simulink model "kamerol"  (R2021b)
settings: Solver=VariableStepAuto  StartTime=0.0  StopTime=10.0  RelTol=1e-3
undefined symbols (not defined in the file): admireDB
libraries: simulink_extras x104, simulink x24, sharedutil x1
(part 13 of 14)

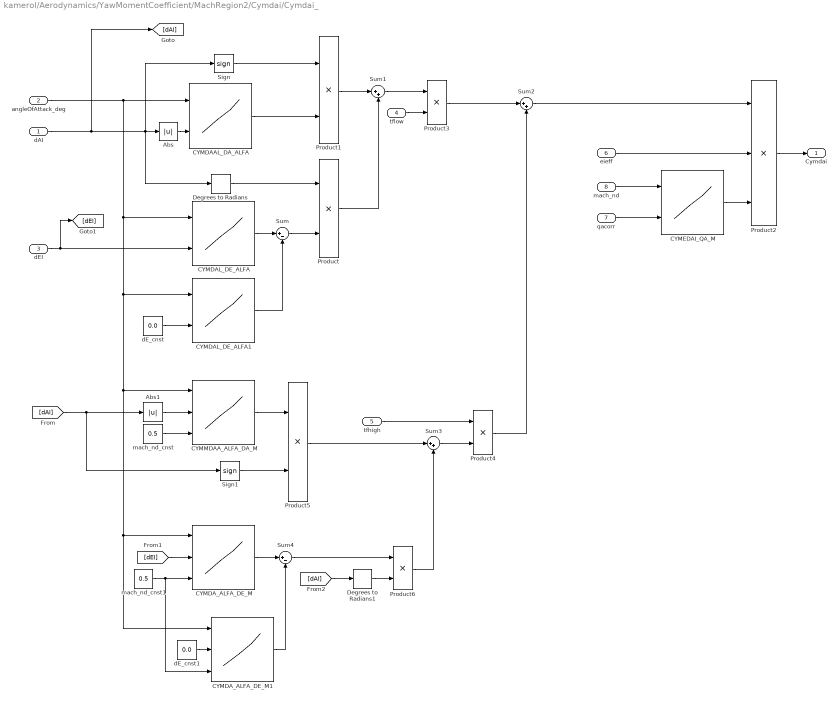
== system kamerol/Aerodynamics/YawMomentCoefficient/MachRegion2/Cymdai/Cymdai_ ==
  dAI : Inport
  angleOfAttack_deg : Inport  Port=2
  dEI : Inport  Port=3
  tflow : Inport  Port=4
  tfhigh : Inport  Port=5
  eieff : Inport  Port=6
  qacorr : Inport  Port=7
  mach_nd : Inport  Port=8
  Abs : Abs
  Abs1 : Abs
  CYMDAAL_DA_ALFA : Lookup_n-D  BreakpointsForDimension1=admireDB.aerodata_asym_ext.CYMDAAL.breakpoints.ALFA  BreakpointsForDimension2=admireDB.aerodata_asym_ext.CYMDAAL.breakpoints.DA  BreakpointsForDimension3=[5, 7]  Table=admireDB.aerodata_asym_ext.CYMDAAL.newTable  ExtrapMethod=Clip  InternalRulePriority=Speed  RndMeth=Simplest  InputSameDT=on
      settings: InputPortMap=u0,u1
  CYMDAL_DE_ALFA : Lookup_n-D  BreakpointsForDimension1=admireDB.aerodata_asym_ext.CYMDAL.breakpoints.ALFA  BreakpointsForDimension2=admireDB.aerodata_asym_ext.CYMDAL.breakpoints.DE  BreakpointsForDimension3=[5, 7]  Table=admireDB.aerodata_asym_ext.CYMDAL.newTable  ExtrapMethod=Clip  InternalRulePriority=Speed  RndMeth=Simplest  InputSameDT=on
      settings: InputPortMap=u0,u1
  CYMDAL_DE_ALFA1 : Lookup_n-D  BreakpointsForDimension1=admireDB.aerodata_asym_ext.CYMDAL.breakpoints.ALFA  BreakpointsForDimension2=admireDB.aerodata_asym_ext.CYMDAL.breakpoints.DE  BreakpointsForDimension3=[5, 7]  Table=admireDB.aerodata_asym_ext.CYMDAL.newTable  ExtrapMethod=Clip  InternalRulePriority=Speed  RndMeth=Simplest  InputSameDT=on
      settings: InputPortMap=u0,u1
  CYMDA_ALFA_DE_M : Lookup_n-D  NumberOfTableDimensions=3  BreakpointsForDimension1=admireDB.aerodata_asym_ext.CYMDA.breakpoints.ALFA  BreakpointsForDimension2=admireDB.aerodata_asym_ext.CYMDA.breakpoints.DE  BreakpointsForDimension3=admireDB.aerodata_asym_ext.CYMDA.breakpoints.M  Table=admireDB.aerodata_asym_ext.CYMDA.newTable  ExtrapMethod=Clip  InternalRulePriority=Speed  RndMeth=Simplest  InputSameDT=on
      settings: InputPortMap=u0,u1,u2
  CYMDA_ALFA_DE_M1 : Lookup_n-D  NumberOfTableDimensions=3  BreakpointsForDimension1=admireDB.aerodata_asym_ext.CYMDA.breakpoints.ALFA  BreakpointsForDimension2=admireDB.aerodata_asym_ext.CYMDA.breakpoints.DE  BreakpointsForDimension3=admireDB.aerodata_asym_ext.CYMDA.breakpoints.M  Table=admireDB.aerodata_asym_ext.CYMDA.newTable  ExtrapMethod=Clip  InternalRulePriority=Speed  RndMeth=Simplest  InputSameDT=on
      settings: InputPortMap=u0,u1,u2
  CYMEDAI_QA_M : Lookup_n-D  BreakpointsForDimension1=admireDB.aerodata_asym_ext.CYMEDAI.breakpoints.M  BreakpointsForDimension2=admireDB.aerodata_asym_ext.CYMEDAI.breakpoints.QA  BreakpointsForDimension3=[5, 7]  Table=admireDB.aerodata_asym_ext.CYMEDAI.newTable  ExtrapMethod=Clip  InternalRulePriority=Speed  RndMeth=Simplest  InputSameDT=on
      settings: InputPortMap=u0,u1
  CYMMDAA_ALFA_DA_M : Lookup_n-D  NumberOfTableDimensions=3  BreakpointsForDimension1=admireDB.aerodata_asym_ext.CYMMDAA.breakpoints.ALFA  BreakpointsForDimension2=admireDB.aerodata_asym_ext.CYMMDAA.breakpoints.DA  BreakpointsForDimension3=admireDB.aerodata_asym_ext.CYMMDAA.breakpoints.M  Table=admireDB.aerodata_asym_ext.CYMMDAA.newTable  ExtrapMethod=Clip  InternalRulePriority=Speed  RndMeth=Simplest  InputSameDT=on
      settings: InputPortMap=u0,u1,u2
  Degrees to Radians : simulink_extras/Transformations/Degrees to Radians
  Degrees to Radians1 : simulink_extras/Transformations/Degrees to Radians
  Product{,1,3..4,6} (5 alike) : Product
  Product2 : Product  Inputs=3
  Product5 : Product  Inputs=**
  Sign : Signum
  Sign1 : Signum
  Sum : Sum  Inputs=|+-
  Sum1 : Sum  Inputs=|++
  Sum2 : Sum  Inputs=|++
  Sum3 : Sum  Inputs=|++
  Sum4 : Sum  Inputs=|+-
  dE_cnst : Constant  Value=0.0
  dE_cnst1 : Constant  Value=0.0
  mach_nd_cnst : Constant  Value=0.5
  mach_nd_cnst1 : Constant  Value=0.5
  Cymdai : Outport
  wires:
  Abs1/1 -> CYMMDAA_ALFA_DA_M/2
  CYMEDAI_QA_M/1 -> Product2/3
  mach_nd/1 -> CYMEDAI_QA_M/1
  qacorr/1 -> CYMEDAI_QA_M/2
  eieff/1 -> Product2/2
  Sum1/1 -> Product3/1
  Product/1 -> Sum1/2
  Product1/1 -> Sum1/1
  Sign/1 -> Product1/1
  CYMDAAL_DA_ALFA/1 -> Product1/2
  Degrees to Radians/1 -> Product/1
  Sum/1 -> Product/2
  CYMDAL_DE_ALFA1/1 -> Sum/2
  CYMDAL_DE_ALFA/1 -> Sum/1
  dEI/1 -> CYMDAL_DE_ALFA/2, [dEI]
  dE_cnst/1 -> CYMDAL_DE_ALFA1/2
  Abs/1 -> CYMDAAL_DA_ALFA/2
  dAI/1 -> [dAI], Sign/1, Abs/1, Degrees to Radians/1
  Product2/1 -> Cymdai/1
  tflow/1 -> Product3/2
  Sum2/1 -> Product2/1
  tfhigh/1 -> Product4/1
  Product3/1 -> Sum2/1
  Product4/1 -> Sum2/2
  angleOfAttack_deg/1 -> CYMDAAL_DA_ALFA/1, CYMDAL_DE_ALFA1/1, CYMDA_ALFA_DE_M1/1, CYMDA_ALFA_DE_M/1, CYMMDAA_ALFA_DA_M/1, CYMDAL_DE_ALFA/1
  mach_nd_cnst/1 -> CYMMDAA_ALFA_DA_M/3
  Sign1/1 -> Product5/2
  [dAI] -> Sign1/1, Abs1/1
  CYMMDAA_ALFA_DA_M/1 -> Product5/1
  Product5/1 -> Sum3/1
  mach_nd_cnst1/1 -> CYMDA_ALFA_DE_M/3, CYMDA_ALFA_DE_M1/3
  [dEI] -> CYMDA_ALFA_DE_M/2
  dE_cnst1/1 -> CYMDA_ALFA_DE_M1/2
  CYMDA_ALFA_DE_M/1 -> Sum4/1
  CYMDA_ALFA_DE_M1/1 -> Sum4/2
  Sum4/1 -> Product6/1
  Degrees to Radians1/1 -> Product6/2
  [dAI] -> Degrees to Radians1/1
  Product6/1 -> Sum3/2
  Sum3/1 -> Product4/2

== system kamerol/Aerodynamics/YawMomentCoefficient/MachRegion2/Cymdaib/Cymdaib_ ==
  angleOfAttack_deg : Inport
  dAI : Inport  Port=2
  angleOfSideslip_deg : Inport  Port=3
  eieff : Inport  Port=4
  tflow : Inport  Port=5
  Abs : Abs
  Abs1 : Abs
  Abs2 : Abs
  CYMDABAL_ALFA : Lookup_n-D  NumberOfTableDimensions=1  BreakpointsForDimension1=admireDB.aerodata_asym_ext.CYMDABAL.breakpoints.ALFA  BreakpointsForDimension3=[5, 7]  Table=admireDB.aerodata_asym_ext.CYMDABAL.newTable  ExtrapMethod=Clip  InternalRulePriority=Speed  RndMeth=Simplest  InputSameDT=on
  Constant : Constant  Value=1/30
  Constant1 : Constant  Value=1/20
  Product : Product  Inputs=*******
  Cymdaib : Outport
  wires:
  eieff/1 -> Product/6
  Abs2/1 -> Product/4
  Constant1/1 -> Product/5
  angleOfSideslip_deg/1 -> Abs2/1
  Constant/1 -> Product/3
  Abs1/1 -> Product/2
  Abs/1 -> CYMDABAL_ALFA/1
  dAI/1 -> Abs1/1
  CYMDABAL_ALFA/1 -> Product/1
  angleOfAttack_deg/1 -> Abs/1
  Product/1 -> Cymdaib/1
  tflow/1 -> Product/7

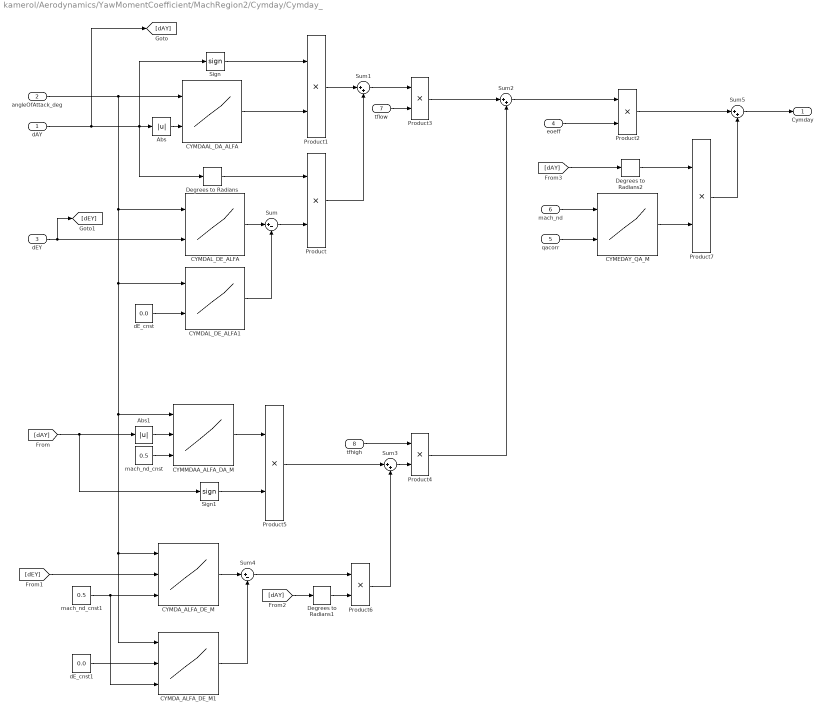
== system kamerol/Aerodynamics/YawMomentCoefficient/MachRegion2/Cymday/Cymday_ ==
  dAY : Inport
  angleOfAttack_deg : Inport  Port=2
  dEY : Inport  Port=3
  eoeff : Inport  Port=4
  qacorr : Inport  Port=5
  mach_nd : Inport  Port=6
  tflow : Inport  Port=7
  tfhigh : Inport  Port=8
  Abs : Abs
  Abs1 : Abs
  CYMDAAL_DA_ALFA : Lookup_n-D  BreakpointsForDimension1=admireDB.aerodata_asym_ext.CYMDAAL.breakpoints.ALFA  BreakpointsForDimension2=admireDB.aerodata_asym_ext.CYMDAAL.breakpoints.DA  BreakpointsForDimension3=[5, 7]  Table=admireDB.aerodata_asym_ext.CYMDAAL.newTable  ExtrapMethod=Clip  InternalRulePriority=Speed  RndMeth=Simplest  InputSameDT=on
      settings: InputPortMap=u0,u1
  CYMDAL_DE_ALFA : Lookup_n-D  BreakpointsForDimension1=admireDB.aerodata_asym_ext.CYMDAL.breakpoints.ALFA  BreakpointsForDimension2=admireDB.aerodata_asym_ext.CYMDAL.breakpoints.DE  BreakpointsForDimension3=[5, 7]  Table=admireDB.aerodata_asym_ext.CYMDAL.newTable  ExtrapMethod=Clip  InternalRulePriority=Speed  RndMeth=Simplest  InputSameDT=on
      settings: InputPortMap=u0,u1
  CYMDAL_DE_ALFA1 : Lookup_n-D  BreakpointsForDimension1=admireDB.aerodata_asym_ext.CYMDAL.breakpoints.ALFA  BreakpointsForDimension2=admireDB.aerodata_asym_ext.CYMDAL.breakpoints.DE  BreakpointsForDimension3=[5, 7]  Table=admireDB.aerodata_asym_ext.CYMDAL.newTable  ExtrapMethod=Clip  InternalRulePriority=Speed  RndMeth=Simplest  InputSameDT=on
      settings: InputPortMap=u0,u1
  CYMDA_ALFA_DE_M : Lookup_n-D  NumberOfTableDimensions=3  BreakpointsForDimension1=admireDB.aerodata_asym_ext.CYMDA.breakpoints.ALFA  BreakpointsForDimension2=admireDB.aerodata_asym_ext.CYMDA.breakpoints.DE  BreakpointsForDimension3=admireDB.aerodata_asym_ext.CYMDA.breakpoints.M  Table=admireDB.aerodata_asym_ext.CYMDA.newTable  ExtrapMethod=Clip  InternalRulePriority=Speed  RndMeth=Simplest  InputSameDT=on
      settings: InputPortMap=u0,u1,u2
  CYMDA_ALFA_DE_M1 : Lookup_n-D  NumberOfTableDimensions=3  BreakpointsForDimension1=admireDB.aerodata_asym_ext.CYMDA.breakpoints.ALFA  BreakpointsForDimension2=admireDB.aerodata_asym_ext.CYMDA.breakpoints.DE  BreakpointsForDimension3=admireDB.aerodata_asym_ext.CYMDA.breakpoints.M  Table=admireDB.aerodata_asym_ext.CYMDA.newTable  ExtrapMethod=Clip  InternalRulePriority=Speed  RndMeth=Simplest  InputSameDT=on
      settings: InputPortMap=u0,u1,u2
  CYMEDAY_QA_M : Lookup_n-D  BreakpointsForDimension1=admireDB.aerodata_asym_ext.CYMEDAY.breakpoints.M  BreakpointsForDimension2=admireDB.aerodata_asym_ext.CYMEDAY.breakpoints.QA  BreakpointsForDimension3=[5, 7]  Table=admireDB.aerodata_asym_ext.CYMEDAY.newTable  ExtrapMethod=Clip  InternalRulePriority=Speed  RndMeth=Simplest  InputSameDT=on
      settings: InputPortMap=u0,u1
  CYMMDAA_ALFA_DA_M : Lookup_n-D  NumberOfTableDimensions=3  BreakpointsForDimension1=admireDB.aerodata_asym_ext.CYMMDAA.breakpoints.ALFA  BreakpointsForDimension2=admireDB.aerodata_asym_ext.CYMMDAA.breakpoints.DA  BreakpointsForDimension3=admireDB.aerodata_asym_ext.CYMMDAA.breakpoints.M  Table=admireDB.aerodata_asym_ext.CYMMDAA.newTable  ExtrapMethod=Clip  InternalRulePriority=Speed  RndMeth=Simplest  InputSameDT=on
      settings: InputPortMap=u0,u1,u2
  Degrees to Radians : simulink_extras/Transformations/Degrees to Radians
  Degrees to Radians1 : simulink_extras/Transformations/Degrees to Radians
  Degrees to Radians2 : simulink_extras/Transformations/Degrees to Radians
  Product{,1..4,6..7} (7 alike) : Product
  Product5 : Product  Inputs=**
  Sign : Signum
  Sign1 : Signum
  Sum : Sum  Inputs=|+-
  Sum{1..3,5} (4 alike) : Sum  Inputs=|++
  Sum4 : Sum  Inputs=|+-
  dE_cnst : Constant  Value=0.0
  dE_cnst1 : Constant  Value=0.0
  mach_nd_cnst : Constant  Value=0.5
  mach_nd_cnst1 : Constant  Value=0.5
  Cymday : Outport
  wires:
  Product7/1 -> Sum5/2
  Product2/1 -> Sum5/1
  Degrees to Radians2/1 -> Product7/1
  [dAY] -> Degrees to Radians2/1
  Sum3/1 -> Product4/2
  Product6/1 -> Sum3/2
  [dAY] -> Degrees to Radians1/1
  Degrees to Radians1/1 -> Product6/2
  Sum4/1 -> Product6/1
  CYMDA_ALFA_DE_M1/1 -> Sum4/2
  CYMDA_ALFA_DE_M/1 -> Sum4/1
  dE_cnst1/1 -> CYMDA_ALFA_DE_M1/2
  [dEY] -> CYMDA_ALFA_DE_M/2
  mach_nd_cnst1/1 -> CYMDA_ALFA_DE_M1/3, CYMDA_ALFA_DE_M/3
  Product5/1 -> Sum3/1
  CYMMDAA_ALFA_DA_M/1 -> Product5/1
  [dAY] -> Abs1/1, Sign1/1
  Sign1/1 -> Product5/2
  mach_nd_cnst/1 -> CYMMDAA_ALFA_DA_M/3
  angleOfAttack_deg/1 -> CYMDAAL_DA_ALFA/1, CYMDAL_DE_ALFA/1, CYMDAL_DE_ALFA1/1, CYMDA_ALFA_DE_M/1, CYMDA_ALFA_DE_M1/1, CYMMDAA_ALFA_DA_M/1
  Product4/1 -> Sum2/2
  Product3/1 -> Sum2/1
  tfhigh/1 -> Product4/1
  Sum2/1 -> Product2/1
  tflow/1 -> Product3/2
  Sum5/1 -> Cymday/1
  dAY/1 -> [dAY], Abs/1, Sign/1, Degrees to Radians/1
  Abs/1 -> CYMDAAL_DA_ALFA/2
  dE_cnst/1 -> CYMDAL_DE_ALFA1/2
  dEY/1 -> CYMDAL_DE_ALFA/2, [dEY]
  CYMDAL_DE_ALFA/1 -> Sum/1
  CYMDAL_DE_ALFA1/1 -> Sum/2
  Sum/1 -> Product/2
  Degrees to Radians/1 -> Product/1
  CYMDAAL_DA_ALFA/1 -> Product1/2
  Sign/1 -> Product1/1
  Product1/1 -> Sum1/1
  Product/1 -> Sum1/2
  Sum1/1 -> Product3/1
  eoeff/1 -> Product2/2
  qacorr/1 -> CYMEDAY_QA_M/2
  mach_nd/1 -> CYMEDAY_QA_M/1
  CYMEDAY_QA_M/1 -> Product7/2
  Abs1/1 -> CYMMDAA_ALFA_DA_M/2

== system kamerol/Aerodynamics/YawMomentCoefficient/MachRegion2/Cymdayb/Cymdayb_ ==
  angleOfAttack_deg : Inport
  dAY : Inport  Port=2
  angleOfSideslip_deg : Inport  Port=3
  eoeff : Inport  Port=4
  tflow : Inport  Port=5
  Abs : Abs
  Abs1 : Abs
  Abs2 : Abs
  CYMDABAL_ALFA : Lookup_n-D  NumberOfTableDimensions=1  BreakpointsForDimension1=admireDB.aerodata_asym_ext.CYMDABAL.breakpoints.ALFA  BreakpointsForDimension3=[5, 7]  Table=admireDB.aerodata_asym_ext.CYMDABAL.newTable  ExtrapMethod=Clip  InternalRulePriority=Speed  RndMeth=Simplest  InputSameDT=on
  Constant : Constant  Value=1/30
  Constant1 : Constant  Value=1/20
  Product : Product  Inputs=*******
  Cymdayb : Outport
  wires:
  Product/1 -> Cymdayb/1
  angleOfAttack_deg/1 -> Abs/1
  CYMDABAL_ALFA/1 -> Product/1
  dAY/1 -> Abs1/1
  Abs/1 -> CYMDABAL_ALFA/1
  Abs1/1 -> Product/2
  Constant/1 -> Product/3
  angleOfSideslip_deg/1 -> Abs2/1
  Constant1/1 -> Product/5
  Abs2/1 -> Product/4
  eoeff/1 -> Product/6
  tflow/1 -> Product/7

== system kamerol/Aerodynamics/YawMomentCoefficient/MachRegion2/Cymdna/Cymdna_ ==
  dNE : Inport
  angleOfAttack_deg : Inport  Port=2
  tflow : Inport  Port=3
  tfhigh : Inport  Port=4
  dNA : Inport  Port=5
  CYMDNAAL_DNE_ALFA : Lookup_n-D  BreakpointsForDimension1=admireDB.aerodata_asym_ext.CYMDNAAL.breakpoints.ALFA  BreakpointsForDimension2=admireDB.aerodata_asym_ext.CYMDNAAL.breakpoints.DNE  BreakpointsForDimension3=[5, 7]  Table=admireDB.aerodata_asym_ext.CYMDNAAL.newTable  ExtrapMethod=Clip  InternalRulePriority=Speed  RndMeth=Simplest  InputSameDT=on
      settings: InputPortMap=u0,u1
  CYMDNAAM_ALFA_M : Lookup_n-D  BreakpointsForDimension1=admireDB.aerodata_asym_ext.CYMDNAAM.breakpoints.M  BreakpointsForDimension2=admireDB.aerodata_asym_ext.CYMDNAAM.breakpoints.ALFA  BreakpointsForDimension3=[5, 7]  Table=admireDB.aerodata_asym_ext.CYMDNAAM.newTable  ExtrapMethod=Clip  InternalRulePriority=Speed  RndMeth=Simplest  InputSameDT=on
      settings: InputPortMap=u0,u1
  Degrees to Radians : simulink_extras/Transformations/Degrees to Radians
  Product : Product  Inputs=**
  Product1 : Product
  Product2 : Product  Inputs=**
  Sum : Sum  Inputs=|++
  mach_nd_cnst : Constant  Value=0.5
  Cymdna : Outport
  wires:
  Degrees to Radians/1 -> Product/2
  CYMDNAAL_DNE_ALFA/1 -> Product1/1
  dNA/1 -> Degrees to Radians/1
  dNE/1 -> CYMDNAAL_DNE_ALFA/2
  angleOfAttack_deg/1 -> CYMDNAAL_DNE_ALFA/1, CYMDNAAM_ALFA_M/2
  Product/1 -> Cymdna/1
  tflow/1 -> Product1/2
  mach_nd_cnst/1 -> CYMDNAAM_ALFA_M/1
  tfhigh/1 -> Product2/2
  CYMDNAAM_ALFA_M/1 -> Product2/1
  Product1/1 -> Sum/1
  Product2/1 -> Sum/2
  Sum/1 -> Product/1

== system kamerol/Aerodynamics/YawMomentCoefficient/MachRegion2/Cymdr/Cymdr_ ==
  angleOfAttack_deg : Inport
  dR : Inport  Port=2
  angleOfSideslip_deg : Inport  Port=3
  tfhigh : Inport  Port=4
  tflow : Inport  Port=5
  qacorr : Inport  Port=6
  mach_nd : Inport  Port=7
  CYMBDRAL_ALFA_DR_BETA : Lookup_n-D  NumberOfTableDimensions=3  BreakpointsForDimension1=admireDB.aerodata_asym_ext.CYMBDRAL.breakpoints.ALFA  BreakpointsForDimension2=admireDB.aerodata_asym_ext.CYMBDRAL.breakpoints.DR  BreakpointsForDimension3=admireDB.aerodata_asym_ext.CYMBDRAL.breakpoints.BETA  Table=admireDB.aerodata_asym_ext.CYMBDRAL.newTable  ExtrapMethod=Clip  InternalRulePriority=Speed  RndMeth=Simplest  InputSameDT=on
      settings: InputPortMap=u0,u1,u2
  CYMDRAM_ALFA_M : Lookup_n-D  BreakpointsForDimension1=admireDB.aerodata_asym_ext.CYMDRAM.breakpoints.M  BreakpointsForDimension2=admireDB.aerodata_asym_ext.CYMDRAM.breakpoints.ALFA  BreakpointsForDimension3=[5, 7]  Table=admireDB.aerodata_asym_ext.CYMDRAM.newTable  ExtrapMethod=Clip  InternalRulePriority=Speed  RndMeth=Simplest  InputSameDT=on
      settings: InputPortMap=u0,u1
  CYMEDR_QA_M : Lookup_n-D  BreakpointsForDimension1=admireDB.aerodata_asym_ext.CYMEDR.breakpoints.M  BreakpointsForDimension2=admireDB.aerodata_asym_ext.CYMEDR.breakpoints.QA  BreakpointsForDimension3=[5, 7]  Table=admireDB.aerodata_asym_ext.CYMEDR.newTable  ExtrapMethod=Clip  InternalRulePriority=Speed  RndMeth=Simplest  InputSameDT=on
      settings: InputPortMap=u0,u1
  Degrees to Radians : simulink_extras/Transformations/Degrees to Radians
  Product : Product
  Product1 : Product  Inputs=***
  Product2 : Product
  Sum : Sum  Inputs=++|
  mach_nd_cnst : Constant  Value=0.5
  Cymdr : Outport
  wires:
  CYMBDRAL_ALFA_DR_BETA/1 -> Product/1
  tflow/1 -> Product/2
  angleOfSideslip_deg/1 -> CYMBDRAL_ALFA_DR_BETA/3
  angleOfAttack_deg/1 -> CYMBDRAL_ALFA_DR_BETA/1, CYMDRAM_ALFA_M/2
  mach_nd/1 -> CYMEDR_QA_M/1
  qacorr/1 -> CYMEDR_QA_M/2
  Product/1 -> Sum/1
  dR/1 -> Degrees to Radians/1, CYMBDRAL_ALFA_DR_BETA/2
  tfhigh/1 -> Product1/3
  mach_nd_cnst/1 -> CYMDRAM_ALFA_M/1
  Degrees to Radians/1 -> Product1/2
  CYMDRAM_ALFA_M/1 -> Product1/1
  Product1/1 -> Sum/2
  Sum/1 -> Product2/1
  CYMEDR_QA_M/1 -> Product2/2
  Product2/1 -> Cymdr/1

== system kamerol/Aerodynamics/YawMomentCoefficient/MachRegion2/Cymp/Cymp_ ==
  dN : Inport
  angleOfAttack_deg : Inport  Port=2
  tflow : Inport  Port=3
  tfhigh : Inport  Port=4
  pc : Inport  Port=5
  qacorr : Inport  Port=6
  mach_nd : Inport  Port=7
  CYMEP_QA_M : Lookup_n-D  BreakpointsForDimension1=admireDB.aerodata_asym_ext.CYMEP.breakpoints.M  BreakpointsForDimension2=admireDB.aerodata_asym_ext.CYMEP.breakpoints.QA  BreakpointsForDimension3=[5, 7]  Table=admireDB.aerodata_asym_ext.CYMEP.newTable  ExtrapMethod=Clip  InternalRulePriority=Speed  RndMeth=Simplest  InputSameDT=on
      settings: InputPortMap=u0,u1
  CYMPAL_DN_ALFA : Lookup_n-D  BreakpointsForDimension1=admireDB.aerodata_asym_ext.CYMPAL.breakpoints.ALFA  BreakpointsForDimension2=admireDB.aerodata_asym_ext.CYMPAL.breakpoints.DN  BreakpointsForDimension3=[5, 7]  Table=admireDB.aerodata_asym_ext.CYMPAL.newTable  ExtrapMethod=Clip  InternalRulePriority=Speed  RndMeth=Simplest  InputSameDT=on
      settings: InputPortMap=u0,u1
  CYMPAM_ALFA_M : Lookup_n-D  BreakpointsForDimension1=admireDB.aerodata_asym_ext.CYMPAM.breakpoints.M  BreakpointsForDimension2=admireDB.aerodata_asym_ext.CYMPAM.breakpoints.ALFA  BreakpointsForDimension3=[5, 7]  Table=admireDB.aerodata_asym_ext.CYMPAM.newTable  ExtrapMethod=Clip  InternalRulePriority=Speed  RndMeth=Simplest  InputSameDT=on
      settings: InputPortMap=u0,u1
  Product : Product  Inputs=3
  Product1 : Product  Inputs=**
  Product2 : Product  Inputs=**
  Sum : Sum  Inputs=|++
  mach_nd_cnst : Constant  Value=0.5
  Cymp : Outport
  wires:
  Product/1 -> Cymp/1
  pc/1 -> Product/2
  CYMEP_QA_M/1 -> Product/3
  CYMPAL_DN_ALFA/1 -> Product1/1
  dN/1 -> CYMPAL_DN_ALFA/2
  angleOfAttack_deg/1 -> CYMPAL_DN_ALFA/1, CYMPAM_ALFA_M/2
  mach_nd/1 -> CYMEP_QA_M/1
  qacorr/1 -> CYMEP_QA_M/2
  mach_nd_cnst/1 -> CYMPAM_ALFA_M/1
  tflow/1 -> Product1/2
  CYMPAM_ALFA_M/1 -> Product2/2
  tfhigh/1 -> Product2/1
  Product1/1 -> Sum/1
  Product2/1 -> Sum/2
  Sum/1 -> Product/1

== system kamerol/Aerodynamics/YawMomentCoefficient/MachRegion2/Cympbeta/Cympbeta_ ==
  angleOfSideslip_deg : Inport
  angleOfAttack_deg : Inport  Port=2
  pc : Inport  Port=3
  tflow : Inport  Port=4
  Abs : Abs
  CYMPBA_BETA_ALFA : Lookup_n-D  BreakpointsForDimension1=admireDB.aerodata_asym_ext.CYMPBA.breakpoints.ALFA  BreakpointsForDimension2=admireDB.aerodata_asym_ext.CYMPBA.breakpoints.BETA  BreakpointsForDimension3=[5, 7]  Table=admireDB.aerodata_asym_ext.CYMPBA.newTable  ExtrapMethod=Clip  InternalRulePriority=Speed  RndMeth=Simplest  InputSameDT=on
      settings: InputPortMap=u0,u1
  Product : Product  Inputs=***
  Cympbeta : Outport
  wires:
  Abs/1 -> CYMPBA_BETA_ALFA/2
  CYMPBA_BETA_ALFA/1 -> Product/1
  angleOfSideslip_deg/1 -> Abs/1
  angleOfAttack_deg/1 -> CYMPBA_BETA_ALFA/1
  pc/1 -> Product/2
  Product/1 -> Cympbeta/1
  tflow/1 -> Product/3

== system kamerol/Aerodynamics/YawMomentCoefficient/MachRegion2/Cymr/Cymr_ ==
  dN : Inport
  angleOfAttack_deg : Inport  Port=2
  tflow : Inport  Port=3
  tfhigh : Inport  Port=4
  rc : Inport  Port=5
  mach_nd : Inport  Port=6
  qacorr : Inport  Port=7
  CYMER_M_QA : Lookup_n-D  BreakpointsForDimension1=admireDB.aerodata_asym_ext.CYMER.breakpoints.QA  BreakpointsForDimension2=admireDB.aerodata_asym_ext.CYMER.breakpoints.M  BreakpointsForDimension3=[5, 7]  Table=admireDB.aerodata_asym_ext.CYMER.newTable  ExtrapMethod=Clip  InternalRulePriority=Speed  RndMeth=Simplest  InputSameDT=on
      settings: InputPortMap=u0,u1
  CYMRAL_DN_ALFA : Lookup_n-D  BreakpointsForDimension1=admireDB.aerodata_asym_ext.CYMRAL.breakpoints.ALFA  BreakpointsForDimension2=admireDB.aerodata_asym_ext.CYMRAL.breakpoints.DN  BreakpointsForDimension3=[5, 7]  Table=admireDB.aerodata_asym_ext.CYMRAL.newTable  ExtrapMethod=Clip  InternalRulePriority=Speed  RndMeth=Simplest  InputSameDT=on
      settings: InputPortMap=u0,u1
  CYMRAM_M_ALFA_DN : Lookup_n-D  NumberOfTableDimensions=3  BreakpointsForDimension1=admireDB.aerodata_asym_ext.CYMRAM.breakpoints.M  BreakpointsForDimension2=admireDB.aerodata_asym_ext.CYMRAM.breakpoints.ALFA  BreakpointsForDimension3=admireDB.aerodata_asym_ext.CYMRAM.breakpoints.DN  Table=admireDB.aerodata_asym_ext.CYMRAM.newTable  ExtrapMethod=Clip  InternalRulePriority=Speed  RndMeth=Simplest  InputSameDT=on
      settings: InputPortMap=u0,u1,u2
  Product : Product  Inputs=***
  Product1 : Product  Inputs=**
  Product2 : Product  Inputs=**
  Sum : Sum  Inputs=|++
  mach_nd_cnst : Constant  Value=0.5
  Cymr : Outport
  wires:
  CYMER_M_QA/1 -> Product/3
  mach_nd/1 -> CYMER_M_QA/2
  qacorr/1 -> CYMER_M_QA/1
  CYMRAL_DN_ALFA/1 -> Product1/1
  dN/1 -> CYMRAM_M_ALFA_DN/3, CYMRAL_DN_ALFA/2
  angleOfAttack_deg/1 -> CYMRAL_DN_ALFA/1, CYMRAM_M_ALFA_DN/2
  Product/1 -> Cymr/1
  rc/1 -> Product/2
  mach_nd_cnst/1 -> CYMRAM_M_ALFA_DN/1
  tflow/1 -> Product1/2
  tfhigh/1 -> Product2/1
  CYMRAM_M_ALFA_DN/1 -> Product2/2
  Product1/1 -> Sum/1
  Product2/1 -> Sum/2
  Sum/1 -> Product/1

== system kamerol/Aerodynamics/YawMomentCoefficient/MachRegion2/Cymrbeta/Cymrbeta_ ==
  angleOfSideslip_deg : Inport
  angleOfAttack_deg : Inport  Port=2
  rc : Inport  Port=3
  tflow : Inport  Port=4
  Abs : Abs
  CYMRBA_BETA_ALFA : Lookup_n-D  BreakpointsForDimension1=admireDB.aerodata_asym_ext.CYMRBA.breakpoints.ALFA  BreakpointsForDimension2=admireDB.aerodata_asym_ext.CYMRBA.breakpoints.BETA  BreakpointsForDimension3=[5, 7]  Table=admireDB.aerodata_asym_ext.CYMRBA.newTable  ExtrapMethod=Clip  InternalRulePriority=Speed  RndMeth=Simplest  InputSameDT=on
      settings: InputPortMap=u0,u1
  Product : Product  Inputs=***
  Cymrbeta : Outport
  wires:
  Abs/1 -> CYMRBA_BETA_ALFA/2
  angleOfSideslip_deg/1 -> Abs/1
  angleOfAttack_deg/1 -> CYMRBA_BETA_ALFA/1
  rc/1 -> Product/2
  Product/1 -> Cymrbeta/1
  CYMRBA_BETA_ALFA/1 -> Product/1
  tflow/1 -> Product/3

== system kamerol/Aerodynamics/YawMomentCoefficient/MachRegion3/Cymbcai/Cymbcai_ ==
  CAI : Inport
  angleOfAttack_deg : Inport  Port=2
  angleOfSideslip_deg : Inport  Port=3
  CYMBCAI_CAI_ALFA : Lookup_n-D  BreakpointsForDimension1=admireDB.aerodata_asym_ext.CYMBCAI.breakpoints.ALFA  BreakpointsForDimension2=admireDB.aerodata_asym_ext.CYMBCAI.breakpoints.CAI  BreakpointsForDimension3=[5, 7]  Table=admireDB.aerodata_asym_ext.CYMBCAI.newTable  ExtrapMethod=Clip  InternalRulePriority=Speed  RndMeth=Simplest  InputSameDT=on
      settings: InputPortMap=u0,u1
  Degrees to Radians : simulink_extras/Transformations/Degrees to Radians
  Product : Product  Inputs=**
  Cymbcai : Outport
  wires:
  Product/1 -> Cymbcai/1
  Degrees to Radians/1 -> Product/2
  angleOfAttack_deg/1 -> CYMBCAI_CAI_ALFA/1
  CYMBCAI_CAI_ALFA/1 -> Product/1
  angleOfSideslip_deg/1 -> Degrees to Radians/1
  CAI/1 -> CYMBCAI_CAI_ALFA/2

== system kamerol/Aerodynamics/YawMomentCoefficient/MachRegion3/Cymbde/Cymbde_ ==
  angleOfAttack_deg : Inport
  dEI : Inport  Port=2
  angleOfSideslip_deg : Inport  Port=3
  dEY : Inport  Port=4
  eieff : Inport  Port=5
  eoeff : Inport  Port=6
  mach_nd : Inport  Port=7
  Abs : Abs
  CYMBKM_M : Lookup_n-D  NumberOfTableDimensions=1  BreakpointsForDimension1=admireDB.aerodata_asym_ext.CYMBKM.breakpoints.M  BreakpointsForDimension3=[5, 7]  Table=admireDB.aerodata_asym_ext.CYMBKM.newTable  ExtrapMethod=Clip  InternalRulePriority=Speed  RndMeth=Simplest  InputSameDT=on
  CYMDEB_ALFA_DE_BETA : Lookup_n-D  NumberOfTableDimensions=3  BreakpointsForDimension1=admireDB.aerodata_asym_ext.CYMDEB.breakpoints.ALFA  BreakpointsForDimension2=admireDB.aerodata_asym_ext.CYMDEB.breakpoints.DE  BreakpointsForDimension3=admireDB.aerodata_asym_ext.CYMDEB.breakpoints.BETA  Table=admireDB.aerodata_asym_ext.CYMDEB.newTable  ExtrapMethod=Clip  InternalRulePriority=Speed  RndMeth=Simplest  InputSameDT=on
      settings: InputPortMap=u0,u1,u2
  CYMDEB_ALFA_DE_BETA1 : Lookup_n-D  NumberOfTableDimensions=3  BreakpointsForDimension1=admireDB.aerodata_asym_ext.CYMDEB.breakpoints.ALFA  BreakpointsForDimension2=admireDB.aerodata_asym_ext.CYMDEB.breakpoints.DE  BreakpointsForDimension3=admireDB.aerodata_asym_ext.CYMDEB.breakpoints.BETA  Table=admireDB.aerodata_asym_ext.CYMDEB.newTable  ExtrapMethod=Clip  InternalRulePriority=Speed  RndMeth=Simplest  InputSameDT=on
      settings: InputPortMap=u0,u1,u2
  Product : Product  Inputs=**
  Product1 : Product  Inputs=**
  Product2 : Product  Inputs=***
  Sign : Signum
  Sum : Sum  Inputs=|++
  Cymbde : Outport
  wires:
  mach_nd/1 -> CYMBKM_M/1
  CYMBKM_M/1 -> Product2/3
  Sign/1 -> Product2/2
  Sum/1 -> Product2/1
  Product1/1 -> Sum/2
  Product/1 -> Sum/1
  eoeff/1 -> Product1/2
  CYMDEB_ALFA_DE_BETA1/1 -> Product1/1
  angleOfAttack_deg/1 -> CYMDEB_ALFA_DE_BETA1/1, CYMDEB_ALFA_DE_BETA/1
  Abs/1 -> CYMDEB_ALFA_DE_BETA1/3, CYMDEB_ALFA_DE_BETA/3
  dEY/1 -> CYMDEB_ALFA_DE_BETA1/2
  eieff/1 -> Product/2
  CYMDEB_ALFA_DE_BETA/1 -> Product/1
  angleOfSideslip_deg/1 -> Sign/1, Abs/1
  dEI/1 -> CYMDEB_ALFA_DE_BETA/2
  Product2/1 -> Cymbde/1

== system kamerol/Aerodynamics/YawMomentCoefficient/MachRegion3/Cymbdle/Cymbdle_ ==
  angleOfAttack_deg : Inport
  dEI : Inport  Port=2
  mach_nd : Inport  Port=3
  dEY : Inport  Port=4
  eieff : Inport  Port=5
  eoeff : Inport  Port=6
  angleOfSideslip_deg : Inport  Port=7
  dLE : Inport  Port=8
  CYMBDLE_ALFA_DE_M : Lookup_n-D  NumberOfTableDimensions=3  BreakpointsForDimension1=admireDB.aerodata_asym_ext.CYMBDLE.breakpoints.ALFA  BreakpointsForDimension2=admireDB.aerodata_asym_ext.CYMBDLE.breakpoints.DE  BreakpointsForDimension3=admireDB.aerodata_asym_ext.CYMBDLE.breakpoints.M  Table=admireDB.aerodata_asym_ext.CYMBDLE.newTable  ExtrapMethod=Clip  InternalRulePriority=Speed  RndMeth=Simplest  InputSameDT=on
      settings: InputPortMap=u0,u1,u2
  CYMBDLE_ALFA_DE_M1 : Lookup_n-D  NumberOfTableDimensions=3  BreakpointsForDimension1=admireDB.aerodata_asym_ext.CYMBDLE.breakpoints.ALFA  BreakpointsForDimension2=admireDB.aerodata_asym_ext.CYMBDLE.breakpoints.DE  BreakpointsForDimension3=admireDB.aerodata_asym_ext.CYMBDLE.breakpoints.M  Table=admireDB.aerodata_asym_ext.CYMBDLE.newTable  ExtrapMethod=Clip  InternalRulePriority=Speed  RndMeth=Simplest  InputSameDT=on
      settings: InputPortMap=u0,u1,u2
  Constant : Constant  Value=1/27
  Degrees to Radians : simulink_extras/Transformations/Degrees to Radians
  Product : Product  Inputs=**
  Product1 : Product  Inputs=**
  Product2 : Product  Inputs=****
  Sum : Sum  Inputs=|++
  Cymbdle : Outport
  wires:
  Constant/1 -> Product2/4
  dLE/1 -> Product2/3
  Degrees to Radians/1 -> Product2/1
  angleOfSideslip_deg/1 -> Degrees to Radians/1
  Sum/1 -> Product2/2
  Product1/1 -> Sum/2
  Product/1 -> Sum/1
  eoeff/1 -> Product1/2
  dEY/1 -> CYMBDLE_ALFA_DE_M1/2
  CYMBDLE_ALFA_DE_M1/1 -> Product1/1
  angleOfAttack_deg/1 -> CYMBDLE_ALFA_DE_M/1, CYMBDLE_ALFA_DE_M1/1
  mach_nd/1 -> CYMBDLE_ALFA_DE_M/3, CYMBDLE_ALFA_DE_M1/3
  eieff/1 -> Product/2
  dEI/1 -> CYMBDLE_ALFA_DE_M/2
  CYMBDLE_ALFA_DE_M/1 -> Product/1
  Product2/1 -> Cymbdle/1

== system kamerol/Aerodynamics/YawMomentCoefficient/MachRegion3/Cymbdn/Cymbdn_ ==
  angleOfAttack_deg : Inport
  dN : Inport  Port=2
  angleOfSideslip_deg : Inport  Port=3
  Abs : Abs
  CYMDNB_ALFA_DN_BETA : Lookup_n-D  NumberOfTableDimensions=3  BreakpointsForDimension1=admireDB.aerodata_asym_ext.CYMDNB.breakpoints.ALFA  BreakpointsForDimension2=admireDB.aerodata_asym_ext.CYMDNB.breakpoints.DN  BreakpointsForDimension3=admireDB.aerodata_asym_ext.CYMDNB.breakpoints.BETA  Table=admireDB.aerodata_asym_ext.CYMDNB.newTable  ExtrapMethod=Clip  InternalRulePriority=Speed  RndMeth=Simplest  InputSameDT=on
      settings: InputPortMap=u0,u1,u2
  Product : Product  Inputs=**
  Sign : Signum
  Cymbdn : Outport
  wires:
  Abs/1 -> CYMDNB_ALFA_DN_BETA/3
  dN/1 -> CYMDNB_ALFA_DN_BETA/2
  CYMDNB_ALFA_DN_BETA/1 -> Product/1
  Sign/1 -> Product/2
  angleOfAttack_deg/1 -> CYMDNB_ALFA_DN_BETA/1
  angleOfSideslip_deg/1 -> Abs/1, Sign/1
  Product/1 -> Cymbdn/1

== system kamerol/Aerodynamics/YawMomentCoefficient/MachRegion3/Cymbeta/Cymbeta_ ==
  angleOfSideslip_deg : Inport
  angleOfAttack_deg : Inport  Port=2
  mach_nd : Inport  Port=3
  qacorr : Inport  Port=4
  Abs : Abs
  CYMEB_QA_M : Lookup_n-D  BreakpointsForDimension1=admireDB.aerodata_asym_ext.CYMEB.breakpoints.M  BreakpointsForDimension2=admireDB.aerodata_asym_ext.CYMEB.breakpoints.QA  BreakpointsForDimension3=[5, 7]  Table=admireDB.aerodata_asym_ext.CYMEB.newTable  ExtrapMethod=Clip  InternalRulePriority=Speed  RndMeth=Simplest  InputSameDT=on
      settings: InputPortMap=u0,u1
  CYMMAB_BETA_ALFA_M : Lookup_n-D  NumberOfTableDimensions=3  BreakpointsForDimension1=admireDB.aerodata_asym_ext.CYMMAB.breakpoints.BETA  BreakpointsForDimension2=admireDB.aerodata_asym_ext.CYMMAB.breakpoints.ALFA  BreakpointsForDimension3=admireDB.aerodata_asym_ext.CYMMAB.breakpoints.M  Table=admireDB.aerodata_asym_ext.CYMMAB.newTable  ExtrapMethod=Clip  InternalRulePriority=Speed  RndMeth=Simplest  InputSameDT=on
      settings: InputPortMap=u0,u1,u2
  Degrees to Radians : simulink_extras/Transformations/Degrees to Radians
  Product : Product  Inputs=**
  Product1 : Product  Inputs=**
  Sign : Signum
  Sum : Sum  Inputs=|++
  Cymbeta : Outport
  wires:
  Product1/1 -> Sum/2
  Abs/1 -> CYMMAB_BETA_ALFA_M/1
  Degrees to Radians/1 -> Product1/2
  qacorr/1 -> CYMEB_QA_M/2
  CYMEB_QA_M/1 -> Product1/1
  mach_nd/1 -> CYMMAB_BETA_ALFA_M/3, CYMEB_QA_M/1
  angleOfSideslip_deg/1 -> Abs/1, Degrees to Radians/1, Sign/1
  Sum/1 -> Cymbeta/1
  Product/1 -> Sum/1
  Sign/1 -> Product/1
  angleOfAttack_deg/1 -> CYMMAB_BETA_ALFA_M/2
  CYMMAB_BETA_ALFA_M/1 -> Product/2

== system kamerol/Aerodynamics/YawMomentCoefficient/MachRegion3/Cymbetad/Cymbetad_ ==
  angleOfAttack_deg : Inport
  mach_nd : Inport  Port=2
  betad : Inport  Port=3
  CYMBDH_ALFA_M : Lookup_n-D  BreakpointsForDimension1=admireDB.aerodata_asym_ext.CYMBDH.breakpoints.M  BreakpointsForDimension2=admireDB.aerodata_asym_ext.CYMBDH.breakpoints.ALFA  BreakpointsForDimension3=[5, 7]  Table=admireDB.aerodata_asym_ext.CYMBDH.newTable  ExtrapMethod=Clip  InternalRulePriority=Speed  RndMeth=Simplest  InputSameDT=on
      settings: InputPortMap=u0,u1
  Product : Product  Inputs=**
  Cymbetad : Outport
  wires:
  betad/1 -> Product/2
  Product/1 -> Cymbetad/1
  mach_nd/1 -> CYMBDH_ALFA_M/1
  angleOfAttack_deg/1 -> CYMBDH_ALFA_M/2
  CYMBDH_ALFA_M/1 -> Product/1

== system kamerol/Aerodynamics/YawMomentCoefficient/MachRegion3/Cymblg/Cymblg_ ==
  angleOfSideslip_deg : Inport
  dLG : Inport  Port=2
  angleOfAttack_deg : Inport  Port=3
  CYMBLST_NG_DOOR_ALFA : Lookup_n-D  BreakpointsForDimension1=admireDB.aerodata_asym_ext.CYMBLST.breakpoints.ALFA  BreakpointsForDimension2=admireDB.aerodata_asym_ext.CYMBLST.breakpoints.NG_DOOR  BreakpointsForDimension3=[5, 7]  Table=admireDB.aerodata_asym_ext.CYMBLST.newTable  ExtrapMethod=Clip  InternalRulePriority=Speed  RndMeth=Simplest  InputSameDT=on
      settings: InputPortMap=u0,u1
  Degrees to Radians : simulink_extras/Transformations/Degrees to Radians
  Product : Product  Inputs=3
  Cymblg : Outport
  wires:
  Degrees to Radians/1 -> Product/1
  angleOfAttack_deg/1 -> CYMBLST_NG_DOOR_ALFA/1
  angleOfSideslip_deg/1 -> Degrees to Radians/1
  dLG/1 -> CYMBLST_NG_DOOR_ALFA/2, Product/2
  Product/1 -> Cymblg/1
  CYMBLST_NG_DOOR_ALFA/1 -> Product/3

== system kamerol/Aerodynamics/YawMomentCoefficient/MachRegion3/Cymdai/Cymdai_ ==
  angleOfAttack_deg : Inport
  dAI : Inport  Port=2
  mach_nd : Inport  Port=3
  dEI : Inport  Port=4
  qacorr : Inport  Port=5
  eieff : Inport  Port=6
  Abs : Abs
  CYMDA_ALFA_DE_M : Lookup_n-D  NumberOfTableDimensions=3  BreakpointsForDimension1=admireDB.aerodata_asym_ext.CYMDA.breakpoints.ALFA  BreakpointsForDimension2=admireDB.aerodata_asym_ext.CYMDA.breakpoints.DE  BreakpointsForDimension3=admireDB.aerodata_asym_ext.CYMDA.breakpoints.M  Table=admireDB.aerodata_asym_ext.CYMDA.newTable  ExtrapMethod=Clip  InternalRulePriority=Speed  RndMeth=Simplest  InputSameDT=on
      settings: InputPortMap=u0,u1,u2
  CYMDA_ALFA_DE_M1 : Lookup_n-D  NumberOfTableDimensions=3  BreakpointsForDimension1=admireDB.aerodata_asym_ext.CYMDA.breakpoints.ALFA  BreakpointsForDimension2=admireDB.aerodata_asym_ext.CYMDA.breakpoints.DE  BreakpointsForDimension3=admireDB.aerodata_asym_ext.CYMDA.breakpoints.M  Table=admireDB.aerodata_asym_ext.CYMDA.newTable  ExtrapMethod=Clip  InternalRulePriority=Speed  RndMeth=Simplest  InputSameDT=on
      settings: InputPortMap=u0,u1,u2
  CYMEDAI_QA_M : Lookup_n-D  BreakpointsForDimension1=admireDB.aerodata_asym_ext.CYMEDAI.breakpoints.M  BreakpointsForDimension2=admireDB.aerodata_asym_ext.CYMEDAI.breakpoints.QA  BreakpointsForDimension3=[5, 7]  Table=admireDB.aerodata_asym_ext.CYMEDAI.newTable  ExtrapMethod=Clip  InternalRulePriority=Speed  RndMeth=Simplest  InputSameDT=on
      settings: InputPortMap=u0,u1
  CYMMDAA_ALFA_DA_M : Lookup_n-D  NumberOfTableDimensions=3  BreakpointsForDimension1=admireDB.aerodata_asym_ext.CYMMDAA.breakpoints.ALFA  BreakpointsForDimension2=admireDB.aerodata_asym_ext.CYMMDAA.breakpoints.DA  BreakpointsForDimension3=admireDB.aerodata_asym_ext.CYMMDAA.breakpoints.M  Table=admireDB.aerodata_asym_ext.CYMMDAA.newTable  ExtrapMethod=Clip  InternalRulePriority=Speed  RndMeth=Simplest  InputSameDT=on
      settings: InputPortMap=u0,u1,u2
  Constant : Constant  Value=0
  Degrees to Radians : simulink_extras/Transformations/Degrees to Radians
  Product : Product  Inputs=**
  Product1 : Product
  Product2 : Product  Inputs=***
  Sign : Signum
  Sum : Sum  Inputs=|+-
  Sum1 : Sum  Inputs=|++
  Cymdai : Outport
  wires:
  Sum1/1 -> Product2/1
  eieff/1 -> Product2/3
  CYMEDAI_QA_M/1 -> Product2/2
  qacorr/1 -> CYMEDAI_QA_M/2
  [mach] -> CYMEDAI_QA_M/1
  Product1/1 -> Sum1/2
  Product/1 -> Sum1/1
  Degrees to Radians/1 -> Product1/1
  Sum/1 -> Product1/2
  CYMDA_ALFA_DE_M1/1 -> Sum/2
  Constant/1 -> CYMDA_ALFA_DE_M1/2
  CYMDA_ALFA_DE_M/1 -> Sum/1
  angleOfAttack_deg/1 -> CYMDA_ALFA_DE_M/1, CYMDA_ALFA_DE_M1/1, CYMMDAA_ALFA_DA_M/1
  mach_nd/1 -> CYMDA_ALFA_DE_M/3, CYMDA_ALFA_DE_M1/3, CYMMDAA_ALFA_DA_M/3, [mach]
  dEI/1 -> CYMDA_ALFA_DE_M/2
  Abs/1 -> CYMMDAA_ALFA_DA_M/2
  dAI/1 -> Abs/1, Sign/1, Degrees to Radians/1
  Sign/1 -> Product/1
  CYMMDAA_ALFA_DA_M/1 -> Product/2
  Product2/1 -> Cymdai/1

== system kamerol/Aerodynamics/YawMomentCoefficient/MachRegion3/Cymday/Cymday_ ==
  angleOfAttack_deg : Inport
  dAY : Inport  Port=2
  mach_nd : Inport  Port=3
  dEY : Inport  Port=4
  eoef : Inport  Port=5
  qacorr : Inport  Port=6
  Abs : Abs
  CYMDA_ALFA_DE_M : Lookup_n-D  NumberOfTableDimensions=3  BreakpointsForDimension1=admireDB.aerodata_asym_ext.CYMDA.breakpoints.ALFA  BreakpointsForDimension2=admireDB.aerodata_asym_ext.CYMDA.breakpoints.DE  BreakpointsForDimension3=admireDB.aerodata_asym_ext.CYMDA.breakpoints.M  Table=admireDB.aerodata_asym_ext.CYMDA.newTable  ExtrapMethod=Clip  InternalRulePriority=Speed  RndMeth=Simplest  InputSameDT=on
      settings: InputPortMap=u0,u1,u2
  CYMDA_ALFA_DE_M1 : Lookup_n-D  NumberOfTableDimensions=3  BreakpointsForDimension1=admireDB.aerodata_asym_ext.CYMDA.breakpoints.ALFA  BreakpointsForDimension2=admireDB.aerodata_asym_ext.CYMDA.breakpoints.DE  BreakpointsForDimension3=admireDB.aerodata_asym_ext.CYMDA.breakpoints.M  Table=admireDB.aerodata_asym_ext.CYMDA.newTable  ExtrapMethod=Clip  InternalRulePriority=Speed  RndMeth=Simplest  InputSameDT=on
      settings: InputPortMap=u0,u1,u2
  CYMEDAY_QA_M : Lookup_n-D  BreakpointsForDimension1=admireDB.aerodata_asym_ext.CYMEDAY.breakpoints.M  BreakpointsForDimension2=admireDB.aerodata_asym_ext.CYMEDAY.breakpoints.QA  BreakpointsForDimension3=[5, 7]  Table=admireDB.aerodata_asym_ext.CYMEDAY.newTable  ExtrapMethod=Clip  InternalRulePriority=Speed  RndMeth=Simplest  InputSameDT=on
      settings: InputPortMap=u0,u1
  CYMMDAA_ALFA_DA_M : Lookup_n-D  NumberOfTableDimensions=3  BreakpointsForDimension1=admireDB.aerodata_asym_ext.CYMMDAA.breakpoints.ALFA  BreakpointsForDimension2=admireDB.aerodata_asym_ext.CYMMDAA.breakpoints.DA  BreakpointsForDimension3=admireDB.aerodata_asym_ext.CYMMDAA.breakpoints.M  Table=admireDB.aerodata_asym_ext.CYMMDAA.newTable  ExtrapMethod=Clip  InternalRulePriority=Speed  RndMeth=Simplest  InputSameDT=on
      settings: InputPortMap=u0,u1,u2
  Constant : Constant  Value=0
  Degrees to Radians : simulink_extras/Transformations/Degrees to Radians
  Product : Product  Inputs=**
  Product1 : Product
  Product2 : Product
  Product3 : Product
  Sign : Signum
  Sum : Sum  Inputs=|+-
  Sum1 : Sum  Inputs=|++
  Sum2 : Sum  Inputs=|++
  Cymday : Outport
  wires:
  Product3/1 -> Sum2/2
  CYMEDAY_QA_M/1 -> Product3/2
  Product2/1 -> Sum2/1
  [dAI_rad] -> Product3/1
  Sum2/1 -> Cymday/1
  CYMMDAA_ALFA_DA_M/1 -> Product/2
  Sign/1 -> Product/1
  dAY/1 -> Abs/1, Sign/1, Degrees to Radians/1
  Abs/1 -> CYMMDAA_ALFA_DA_M/2
  dEY/1 -> CYMDA_ALFA_DE_M/2
  mach_nd/1 -> CYMDA_ALFA_DE_M1/3, CYMDA_ALFA_DE_M/3, CYMMDAA_ALFA_DA_M/3, [mach]
  angleOfAttack_deg/1 -> CYMMDAA_ALFA_DA_M/1, CYMDA_ALFA_DE_M/1, CYMDA_ALFA_DE_M1/1
  CYMDA_ALFA_DE_M/1 -> Sum/1
  Constant/1 -> CYMDA_ALFA_DE_M1/2
  CYMDA_ALFA_DE_M1/1 -> Sum/2
  Sum/1 -> Product1/2
  Degrees to Radians/1 -> [dAI_rad], Product1/1
  Product/1 -> Sum1/1
  Product1/1 -> Sum1/2
  [mach] -> CYMEDAY_QA_M/1
  qacorr/1 -> CYMEDAY_QA_M/2
  eoef/1 -> Product2/2
  Sum1/1 -> Product2/1

== system kamerol/Aerodynamics/YawMomentCoefficient/MachRegion3/Cymdna/Cymdna_ ==
  angleOfAttack_deg : Inport
  mach_nd : Inport  Port=2
  dNA : Inport  Port=3
  CYMDNAAM_ALFA_M : Lookup_n-D  BreakpointsForDimension1=admireDB.aerodata_asym_ext.CYMDNAAM.breakpoints.M  BreakpointsForDimension2=admireDB.aerodata_asym_ext.CYMDNAAM.breakpoints.ALFA  BreakpointsForDimension3=[5, 7]  Table=admireDB.aerodata_asym_ext.CYMDNAAM.newTable  ExtrapMethod=Clip  InternalRulePriority=Speed  RndMeth=Simplest  InputSameDT=on
      settings: InputPortMap=u0,u1
  Degrees to Radians : simulink_extras/Transformations/Degrees to Radians
  Product : Product  Inputs=**
  Cymdna : Outport
  wires:
  Product/1 -> Cymdna/1
  dNA/1 -> Degrees to Radians/1
  mach_nd/1 -> CYMDNAAM_ALFA_M/1
  Degrees to Radians/1 -> Product/2
  angleOfAttack_deg/1 -> CYMDNAAM_ALFA_M/2
  CYMDNAAM_ALFA_M/1 -> Product/1

== system kamerol/Aerodynamics/YawMomentCoefficient/MachRegion3/Cymdr/Cymdr_ ==
  angleOfAttack_deg : Inport
  mach_nd : Inport  Port=2
  dR : Inport  Port=3
  qacorr : Inport  Port=4
  CYMDRAM_ALFA_M : Lookup_n-D  BreakpointsForDimension1=admireDB.aerodata_asym_ext.CYMDRAM.breakpoints.M  BreakpointsForDimension2=admireDB.aerodata_asym_ext.CYMDRAM.breakpoints.ALFA  BreakpointsForDimension3=[5, 7]  Table=admireDB.aerodata_asym_ext.CYMDRAM.newTable  ExtrapMethod=Clip  InternalRulePriority=Speed  RndMeth=Simplest  InputSameDT=on
      settings: InputPortMap=u0,u1
  CYMEDR_QA_M : Lookup_n-D  BreakpointsForDimension1=admireDB.aerodata_asym_ext.CYMEDR.breakpoints.M  BreakpointsForDimension2=admireDB.aerodata_asym_ext.CYMEDR.breakpoints.QA  BreakpointsForDimension3=[5, 7]  Table=admireDB.aerodata_asym_ext.CYMEDR.newTable  ExtrapMethod=Clip  InternalRulePriority=Speed  RndMeth=Simplest  InputSameDT=on
      settings: InputPortMap=u0,u1
  Degrees to Radians : simulink_extras/Transformations/Degrees to Radians
  Product : Product  Inputs=***
  Cymdr : Outport
  wires:
  Product/1 -> Cymdr/1
  CYMEDR_QA_M/1 -> Product/3
  qacorr/1 -> CYMEDR_QA_M/2
  mach_nd/1 -> CYMEDR_QA_M/1, CYMDRAM_ALFA_M/1
  Degrees to Radians/1 -> Product/2
  angleOfAttack_deg/1 -> CYMDRAM_ALFA_M/2
  CYMDRAM_ALFA_M/1 -> Product/1
  dR/1 -> Degrees to Radians/1

== system kamerol/Aerodynamics/YawMomentCoefficient/MachRegion3/Cymp/Cymp_ ==
  angleOfAttack_deg : Inport
  mach_nd : Inport  Port=2
  qacorr : Inport  Port=3
  pc : Inport  Port=4
  CYMEP_QA_M : Lookup_n-D  BreakpointsForDimension1=admireDB.aerodata_asym_ext.CYMEP.breakpoints.M  BreakpointsForDimension2=admireDB.aerodata_asym_ext.CYMEP.breakpoints.QA  BreakpointsForDimension3=[5, 7]  Table=admireDB.aerodata_asym_ext.CYMEP.newTable  ExtrapMethod=Clip  InternalRulePriority=Speed  RndMeth=Simplest  InputSameDT=on
      settings: InputPortMap=u0,u1
  CYMPAM_ALFA_M : Lookup_n-D  BreakpointsForDimension1=admireDB.aerodata_asym_ext.CYMPAM.breakpoints.M  BreakpointsForDimension2=admireDB.aerodata_asym_ext.CYMPAM.breakpoints.ALFA  BreakpointsForDimension3=[5, 7]  Table=admireDB.aerodata_asym_ext.CYMPAM.newTable  ExtrapMethod=Clip  InternalRulePriority=Speed  RndMeth=Simplest  InputSameDT=on
      settings: InputPortMap=u0,u1
  Product : Product
  Sum : Sum  Inputs=|++
  Cymp : Outport
  wires:
  qacorr/1 -> CYMEP_QA_M/2
  CYMEP_QA_M/1 -> Sum/2
  Sum/1 -> Product/1
  mach_nd/1 -> CYMPAM_ALFA_M/1, CYMEP_QA_M/1
  pc/1 -> Product/2
  Product/1 -> Cymp/1
  angleOfAttack_deg/1 -> CYMPAM_ALFA_M/2
  CYMPAM_ALFA_M/1 -> Sum/1

== system kamerol/Aerodynamics/YawMomentCoefficient/MachRegion3/Cymr/Cymr_ ==
  mach_nd : Inport
  angleOfAttack_deg : Inport  Port=2
  dN : Inport  Port=3
  qacorr : Inport  Port=4
  rc : Inport  Port=5
  CYMER_M_QA : Lookup_n-D  BreakpointsForDimension1=admireDB.aerodata_asym_ext.CYMER.breakpoints.QA  BreakpointsForDimension2=admireDB.aerodata_asym_ext.CYMER.breakpoints.M  BreakpointsForDimension3=[5, 7]  Table=admireDB.aerodata_asym_ext.CYMER.newTable  ExtrapMethod=Clip  InternalRulePriority=Speed  RndMeth=Simplest  InputSameDT=on
      settings: InputPortMap=u0,u1
  CYMRAM_M_ALFA_DN : Lookup_n-D  NumberOfTableDimensions=3  BreakpointsForDimension1=admireDB.aerodata_asym_ext.CYMRAM.breakpoints.M  BreakpointsForDimension2=admireDB.aerodata_asym_ext.CYMRAM.breakpoints.ALFA  BreakpointsForDimension3=admireDB.aerodata_asym_ext.CYMRAM.breakpoints.DN  Table=admireDB.aerodata_asym_ext.CYMRAM.newTable  ExtrapMethod=Clip  InternalRulePriority=Speed  RndMeth=Simplest  InputSameDT=on
      settings: InputPortMap=u0,u1,u2
  Product : Product  Inputs=***
  Cymr : Outport
  wires:
  CYMER_M_QA/1 -> Product/3
  qacorr/1 -> CYMER_M_QA/1
  dN/1 -> CYMRAM_M_ALFA_DN/3
  rc/1 -> Product/2
  Product/1 -> Cymr/1
  mach_nd/1 -> CYMRAM_M_ALFA_DN/1, CYMER_M_QA/2
  angleOfAttack_deg/1 -> CYMRAM_M_ALFA_DN/2
  CYMRAM_M_ALFA_DN/1 -> Product/1

== system kamerol/Aerodynamics/YawMomentCoefficient/MachRegion4/Cymbcai/Cymbcai_ ==
  CAI : Inport
  angleOfAttack_deg : Inport  Port=2
  angleOfSideslip_deg : Inport  Port=3
  CYMBCAI_CAI_ALFA : Lookup_n-D  BreakpointsForDimension1=admireDB.aerodata_asym_ext.CYMBCAI.breakpoints.ALFA  BreakpointsForDimension2=admireDB.aerodata_asym_ext.CYMBCAI.breakpoints.CAI  BreakpointsForDimension3=[5, 7]  Table=admireDB.aerodata_asym_ext.CYMBCAI.newTable  ExtrapMethod=Clip  InternalRulePriority=Speed  RndMeth=Simplest  InputSameDT=on
      settings: InputPortMap=u0,u1
  Degrees to Radians : simulink_extras/Transformations/Degrees to Radians
  Product : Product  Inputs=**
  Cymbcai : Outport
  wires:
  CAI/1 -> CYMBCAI_CAI_ALFA/2
  angleOfSideslip_deg/1 -> Degrees to Radians/1
  CYMBCAI_CAI_ALFA/1 -> Product/1
  angleOfAttack_deg/1 -> CYMBCAI_CAI_ALFA/1
  Degrees to Radians/1 -> Product/2
  Product/1 -> Cymbcai/1

== system kamerol/Aerodynamics/YawMomentCoefficient/MachRegion4/Cymbde/Cymbde_ ==
  angleOfAttack_deg : Inport
  dEI : Inport  Port=2
  angleOfSideslip_deg : Inport  Port=3
  dEY : Inport  Port=4
  eieff : Inport  Port=5
  eoeff : Inport  Port=6
  mach_nd : Inport  Port=7
  Abs : Abs
  CYMBKM_M : Lookup_n-D  NumberOfTableDimensions=1  BreakpointsForDimension1=admireDB.aerodata_asym_ext.CYMBKM.breakpoints.M  BreakpointsForDimension3=[5, 7]  Table=admireDB.aerodata_asym_ext.CYMBKM.newTable  ExtrapMethod=Clip  InternalRulePriority=Speed  RndMeth=Simplest  InputSameDT=on
  CYMDEB_ALFA_DE_BETA : Lookup_n-D  NumberOfTableDimensions=3  BreakpointsForDimension1=admireDB.aerodata_asym_ext.CYMDEB.breakpoints.ALFA  BreakpointsForDimension2=admireDB.aerodata_asym_ext.CYMDEB.breakpoints.DE  BreakpointsForDimension3=admireDB.aerodata_asym_ext.CYMDEB.breakpoints.BETA  Table=admireDB.aerodata_asym_ext.CYMDEB.newTable  ExtrapMethod=Clip  InternalRulePriority=Speed  RndMeth=Simplest  InputSameDT=on
      settings: InputPortMap=u0,u1,u2
  CYMDEB_ALFA_DE_BETA1 : Lookup_n-D  NumberOfTableDimensions=3  BreakpointsForDimension1=admireDB.aerodata_asym_ext.CYMDEB.breakpoints.ALFA  BreakpointsForDimension2=admireDB.aerodata_asym_ext.CYMDEB.breakpoints.DE  BreakpointsForDimension3=admireDB.aerodata_asym_ext.CYMDEB.breakpoints.BETA  Table=admireDB.aerodata_asym_ext.CYMDEB.newTable  ExtrapMethod=Clip  InternalRulePriority=Speed  RndMeth=Simplest  InputSameDT=on
      settings: InputPortMap=u0,u1,u2
  Product : Product  Inputs=**
  Product1 : Product  Inputs=**
  Product2 : Product  Inputs=***
  Sign : Signum
  Sum : Sum  Inputs=|++
  Cymbde : Outport
  wires:
  Product2/1 -> Cymbde/1
  dEI/1 -> CYMDEB_ALFA_DE_BETA/2
  angleOfSideslip_deg/1 -> Abs/1, Sign/1
  CYMDEB_ALFA_DE_BETA/1 -> Product/1
  eieff/1 -> Product/2
  dEY/1 -> CYMDEB_ALFA_DE_BETA1/2
  Abs/1 -> CYMDEB_ALFA_DE_BETA/3, CYMDEB_ALFA_DE_BETA1/3
  angleOfAttack_deg/1 -> CYMDEB_ALFA_DE_BETA/1, CYMDEB_ALFA_DE_BETA1/1
  CYMDEB_ALFA_DE_BETA1/1 -> Product1/1
  eoeff/1 -> Product1/2
  Product/1 -> Sum/1
  Product1/1 -> Sum/2
  Sum/1 -> Product2/1
  Sign/1 -> Product2/2
  CYMBKM_M/1 -> Product2/3
  mach_nd/1 -> CYMBKM_M/1

== system kamerol/Aerodynamics/YawMomentCoefficient/MachRegion4/Cymbdle/Cymbdle_ ==
  angleOfAttack_deg : Inport
  dEI : Inport  Port=2
  mach_nd : Inport  Port=3
  dEY : Inport  Port=4
  eieff : Inport  Port=5
  eoeff : Inport  Port=6
  angleOfSideslip_deg : Inport  Port=7
  dLE : Inport  Port=8
  CYMBDLE_ALFA_DE_M : Lookup_n-D  NumberOfTableDimensions=3  BreakpointsForDimension1=admireDB.aerodata_asym_ext.CYMBDLE.breakpoints.ALFA  BreakpointsForDimension2=admireDB.aerodata_asym_ext.CYMBDLE.breakpoints.DE  BreakpointsForDimension3=admireDB.aerodata_asym_ext.CYMBDLE.breakpoints.M  Table=admireDB.aerodata_asym_ext.CYMBDLE.newTable  ExtrapMethod=Clip  InternalRulePriority=Speed  RndMeth=Simplest  InputSameDT=on
      settings: InputPortMap=u0,u1,u2
  CYMBDLE_ALFA_DE_M1 : Lookup_n-D  NumberOfTableDimensions=3  BreakpointsForDimension1=admireDB.aerodata_asym_ext.CYMBDLE.breakpoints.ALFA  BreakpointsForDimension2=admireDB.aerodata_asym_ext.CYMBDLE.breakpoints.DE  BreakpointsForDimension3=admireDB.aerodata_asym_ext.CYMBDLE.breakpoints.M  Table=admireDB.aerodata_asym_ext.CYMBDLE.newTable  ExtrapMethod=Clip  InternalRulePriority=Speed  RndMeth=Simplest  InputSameDT=on
      settings: InputPortMap=u0,u1,u2
  Constant : Constant  Value=1/27
  Degrees to Radians : simulink_extras/Transformations/Degrees to Radians
  Product : Product  Inputs=**
  Product1 : Product  Inputs=**
  Product2 : Product  Inputs=****
  Sum : Sum  Inputs=|++
  Cymbdle : Outport
  wires:
  Product2/1 -> Cymbdle/1
  CYMBDLE_ALFA_DE_M/1 -> Product/1
  dEI/1 -> CYMBDLE_ALFA_DE_M/2
  eieff/1 -> Product/2
  mach_nd/1 -> CYMBDLE_ALFA_DE_M1/3, CYMBDLE_ALFA_DE_M/3
  angleOfAttack_deg/1 -> CYMBDLE_ALFA_DE_M1/1, CYMBDLE_ALFA_DE_M/1
  CYMBDLE_ALFA_DE_M1/1 -> Product1/1
  dEY/1 -> CYMBDLE_ALFA_DE_M1/2
  eoeff/1 -> Product1/2
  Product/1 -> Sum/1
  Product1/1 -> Sum/2
  Sum/1 -> Product2/2
  angleOfSideslip_deg/1 -> Degrees to Radians/1
  Degrees to Radians/1 -> Product2/1
  dLE/1 -> Product2/3
  Constant/1 -> Product2/4

== system kamerol/Aerodynamics/YawMomentCoefficient/MachRegion4/Cymbdn/Cymbdn_ ==
  angleOfAttack_deg : Inport
  dN : Inport  Port=2
  angleOfSideslip_deg : Inport  Port=3
  Abs : Abs
  CYMDNB_ALFA_DN_BETA : Lookup_n-D  NumberOfTableDimensions=3  BreakpointsForDimension1=admireDB.aerodata_asym_ext.CYMDNB.breakpoints.ALFA  BreakpointsForDimension2=admireDB.aerodata_asym_ext.CYMDNB.breakpoints.DN  BreakpointsForDimension3=admireDB.aerodata_asym_ext.CYMDNB.breakpoints.BETA  Table=admireDB.aerodata_asym_ext.CYMDNB.newTable  ExtrapMethod=Clip  InternalRulePriority=Speed  RndMeth=Simplest  InputSameDT=on
      settings: InputPortMap=u0,u1,u2
  Product : Product  Inputs=**
  Sign : Signum
  Cymbdn : Outport
  wires:
  Product/1 -> Cymbdn/1
  angleOfSideslip_deg/1 -> Sign/1, Abs/1
  angleOfAttack_deg/1 -> CYMDNB_ALFA_DN_BETA/1
  Sign/1 -> Product/2
  CYMDNB_ALFA_DN_BETA/1 -> Product/1
  dN/1 -> CYMDNB_ALFA_DN_BETA/2
  Abs/1 -> CYMDNB_ALFA_DN_BETA/3
